simulink model "calculate_pid"  (R2018b)
settings: Solver=FixedStepDiscrete  StartTime=0.0  StopTime=10.0  RelTol=1e-3
undefined symbols (not defined in the file or in its folder): DiscIntNeverNeededParam
libraries: simulink x1
settings Model: Creator=matlab  LastModifiedBy=matlab
settings DataIOCC: SaveOutput=off  SignalLogging=off  SaveTime=off
settings OptimizationCC: DefaultParameterBehavior=Inlined  EnhancedBackFolding=on  PassReuseOutputArgsAs=Individual arguments  OptimizeBlockOrder=speed  DifferentSizesBufferReuse=on  OptimizationCustomize=off
settings DebuggingCC: ParameterTunabilityLossMsg=error
settings SFSimCC: MATLABDynamicMemAlloc=off
settings RTWCC: SystemTargetFile=ert.tlc  TemplateMakefile=ert_default_tmf  PostCodeGenCommand=packNGo(buildInfo);  GenerateReport=on  IncludeHyperlinkInReport=on  LaunchReport=on  GenerateTraceInfo=on  GenerateTraceReport=on  GenerateTraceReportSl=on  GenerateTraceReportSf=on  GenerateTraceReportEml=on
settings CodeAppCC: ForceParamTrailComments=on  IgnoreCustomStorageClasses=off  OperatorAnnotations=on  SimulinkDataObjDesc=on  SFDataObjDesc=on  InsertBlockDesc=on
settings ERTTargetCC: TargetLangStandard=C99 (ISO)  GenerateSampleERTMain=on  InlinedParameterPlacement=NonHierarchical  ERTCustomFileTemplate=example_file_process.tlc

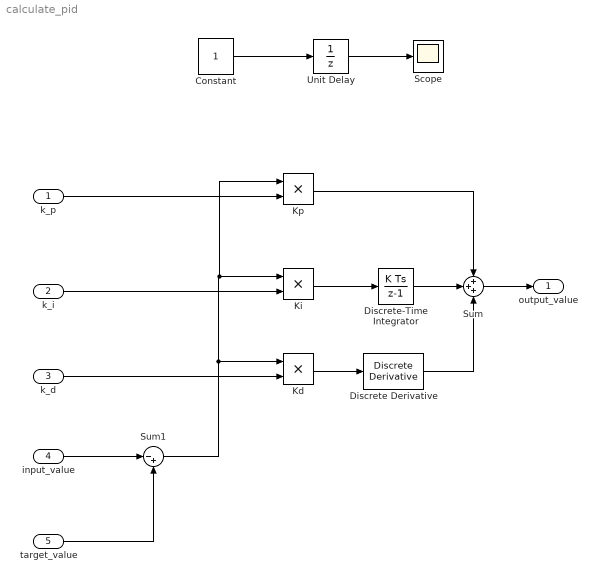
== system calculate_pid ==
  k_p : Inport  OutDataTypeStr=AuroraPIDValue  BusOutputAsStruct=on
  k_i : Inport  Port=2  OutDataTypeStr=AuroraPIDValue  BusOutputAsStruct=on
  k_d : Inport  Port=3  OutDataTypeStr=AuroraPIDValue  BusOutputAsStruct=on
  input_value : Inport  Port=4  OutDataTypeStr=AuroraReal  BusOutputAsStruct=on
  target_value : Inport  Port=5  OutDataTypeStr=AuroraReal  BusOutputAsStruct=on
  Constant : Constant
  Discrete Derivative : simulink/Discrete/Discrete Derivative  gainval=1.0  ICPrevScaledInput=0.0  OutMin=[]  OutMax=[]  OutDataType=fixdt(1, 16)  OutScaling=2^-10  DoSatur=off
  Discrete-Time Integrator : DiscreteIntegrator  SampleTime=-1  ICPrevOutput=DiscIntNeverNeededParam  ICPrevScaledInput=DiscIntNeverNeededParam
  Kd : Product
  Ki : Product
  Kp : Product
  Scope : Scope
  Sum : Sum  Inputs=+++
  Sum1 : Sum  Inputs=|-+
  Unit Delay : UnitDelay  SampleTime=-1
  output_value : Outport  OutDataTypeStr=AuroraPWM
  wires:
  Constant/1 -> Unit Delay/1
  Unit Delay/1 -> Scope/1
  Kd/1 -> Discrete Derivative/1
  Discrete Derivative/1 -> Sum/3
  Sum1/1 -> Ki/1, Kp/1, Kd/1
  Ki/1 -> Discrete-Time Integrator/1
  Discrete-Time Integrator/1 -> Sum/2
  Kp/1 -> Sum/1
  k_p/1 -> Kp/2
  k_i/1 -> Ki/2
  k_d/1 -> Kd/2
  input_value/1 -> Sum1/1
  target_value/1 -> Sum1/2
  Sum/1 -> output_value/1
